simulink model "sdrzfreqcalib_rx"  (R2016a)
settings: Solver=FixedStepDiscrete  StartTime=0.0  StopTime=inf  RelTol=1e-3
libraries: sdrzblksprivate x1, dspspect3 x1, sdrzlib x1
Description:
  | This model is used to calculate the frequency offset between a transmitter and the SDR receiver.
settings Model: ModifiedByFormat=The MathWorks Inc.  SimulationMode=accelerator  Creator=The MathWorks, Inc.  LastModifiedBy=The MathWorks Inc.
settings DataIOCC: LimitDataPoints=on  SaveFormat=Array
settings OptimizationCC: ExpressionDepthLimit=2147483647
settings DebuggingCC: UnderspecifiedInitializationDetection=Classic  MergeDetectMultiDrivingBlocksExec=none  SolverPrmCheckMsg=warning  ParameterPrecisionLossMsg=none  FcnCallInpInsideContextMsg=EnableAllAsWarning  AllowSymbolicDim=off  StateNameClashWarn=warning
settings HardwareCC: ProdBitPerPointer=32  ProdLargestAtomicFloat=None  ProdIntDivRoundTo=Undefined  ProdEndianess=Unspecified  ProdWordSize=32  ProdHWDeviceType=32-bit Generic  TargetBitPerPointer=64  TargetLongLongMode=on  TargetIntDivRoundTo=Zero  TargetEndianess=LittleEndian  TargetWordSize=64  TargetHWDeviceType=Generic->MATLAB Host Computer  ProdEqTarget=off
settings ModelReferenceCC: PropagateSignalLabelsOutOfModel=off
settings RTWCC: CustomSourceCode=|
  | #include<stdio.h>
  | #include<stdlib.h>
settings GRTTargetCC: CombineOutputUpdateFcns=off  GRTInterface=on
settings ConfigComp: CovModelRefEnable=Off  CovSFcnEnable=off

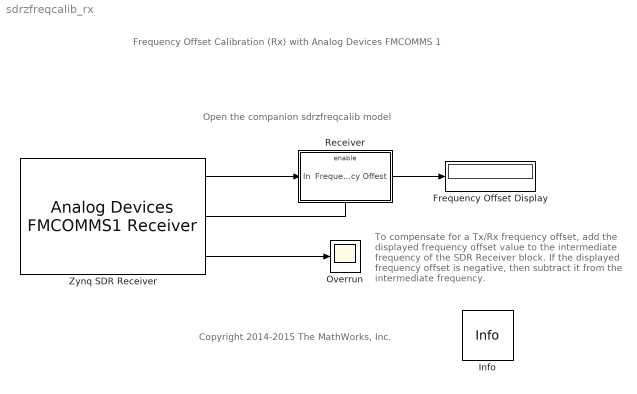
== system sdrzfreqcalib_rx ==
  note: Frequency Offset Calibration (Rx)
      | with Analog Devices FMCOMMS 1
  note: Open the companion sdrzfreqcalib model
  note: Copyright 2014-2015 The MathWorks, Inc.
  note: To compensate for a Tx/Rx frequency offset,
      | add the displayed frequency offset value to the
      | intermediate frequency of the SDR Receiver block. If
      | the displayed frequency offset is negative, then
      | subtract it from the intermediate frequency.
  Frequency Offset Display : Display
  Info : sdrzblksprivate/Info  SystemSampleTime=-1
  Overrun : Scope
  Receiver : Subsystem
      mask Display: disp('Receiver')
  Zynq SDR Receiver : sdrzlib/Analog Devices FMCOMMS1 Receiver  SourceLibraryInfo="This block requires Communications System Toolbox Support Package for Xilinx FPGA-Based Radio. <a href=\"http://www.mathworks.com/hardware-support-packages\">More information</a>"  sobjType=comm.SDRZynqFMCOMMS1Receiver  IPAddress=192.168.3.2  dataUDPPort=-1  ctrlUDPPort=-1  subDeviceList=comm.SDRZynqFMCOMMS1Receiver  sdrBlockType=SDRBlockTypeSLT.SDRRxBlock  requester=UNUSED_BY_SFCN  sdrExecutionMode=HW  LostSamplesOutputPort=on  OutputDataType=double  FrameLength=4096  EnableBurstMode=off  NumFramesInBurst=20  BypassUserLogic=on  DecimatorSelect=DDC decimator  SourceSelect=RF data  SineAmplitude=16000  SineFrequency=30000  EnableInternalClock=off  BypassIQBalance=on  CenterFrequencySource=Dialog  CenterFrequency=2.415e9 - 3e6  IntermediateFrequencySource=Dialog  IntermediateFrequency=3e6  IFBandwidthSource=Dialog  IFBandwidth=40e6  ADCRateSource=Dialog  ADCRate=98.304e6  GainSource=Dialog  Gain=4.5  DecimationFactorSource=Dialog  DecimationFactor=500  RFFrequencyIsTunable=logical(0)  SampleTime=1/(98.304e6/500)  BypassDCBlockingFilter=off  IQBalanceCoefficients=64  SkipAllHardwareResetAndInitialization=off  EnableIQCalibrationTable=on  CacheIQCalibrationTable=off
  wires:
  Zynq SDR Receiver/1 -> Receiver/1(In)
  Zynq SDR Receiver/2 -> Receiver/Enable
  Zynq SDR Receiver/3 -> Overrun/1
  Receiver/1(Frequency Offest) -> Frequency Offset Display/1

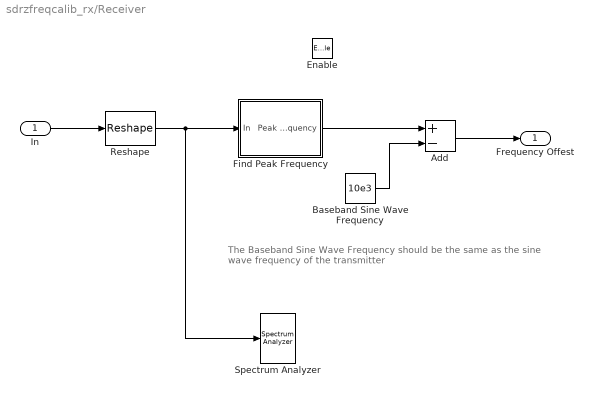
== system sdrzfreqcalib_rx/Receiver ==
  note: The Baseband Sine Wave Frequency should be the same as
      | the sine wave frequency of the transmitter
  In : Inport
  Enable : EnablePort
  Add : Sum  Inputs=+-
  Baseband Sine Wave Frequency : Constant  Value=10e3
  Find Peak Frequency : Subsystem
      mask Display: disp('Find Peak\nFrequency')
  Reshape : Reshape  OutputDimensionality=Customize  OutputDimensions=[4096,1]
  Spectrum Analyzer : SpectrumAnalyzer
  Frequency Offest : Outport
  wires:
  In/1 -> Reshape/1
  Reshape/1 -> Find Peak Frequency/1(In), Spectrum Analyzer/1
  Find Peak Frequency/1(Peak Frequency) -> Add/1
  Baseband Sine Wave Frequency/1 -> Add/2
  Add/1 -> Frequency Offest/1

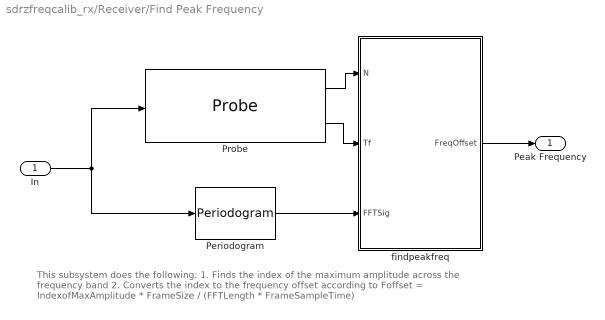
== system sdrzfreqcalib_rx/Receiver/Find Peak Frequency ==
  note: This subsystem does the following:
      | 1.  Finds the index of the maximum amplitude across the frequency band
      | 2.  Converts the index to the frequency offset according to
      | Foffset = IndexofMaxAmplitude * FrameSize / (FFTLength * FrameSampleTime)
  In : Inport
  Periodogram : dspspect3/Periodogram  measurement=Power spectral density  wintype=Hamming  Rs=50  beta=5  winsamp=Symmetric  FFTImplementation=Auto  inheritFFT=off  fftsize=4096  navg=2  inheritTs=on  Ts=1
  Probe : Probe  ProbeComplexSignal=off
  findpeakfreq : MATLAB Function  TreatAsAtomicUnit=on
  Peak Frequency : Outport
  wires:
  Periodogram/1 -> findpeakfreq/3(FFTSig)
  Probe/1 -> findpeakfreq/1(N)
  Probe/2 -> findpeakfreq/2(Tf)
  findpeakfreq/1(FreqOffset) -> Peak Frequency/1
  In/1 -> Periodogram/1, Probe/1

== matlab function sdrzfreqcalib_rx/Receiver/Find Peak Frequency/findpeakfreq ==
  data: N input; FreqOffset output; Tf input; FFTSig input
function FreqOffset  = findpeakfreq(N, Tf, FFTSig)
% Find peak frequency
% N - frame size
% Tf - frame sample time
% FFTSig - result of FFT

%#codegen

FFTSize = length(FFTSig);
FFTSig = fftshift(FFTSig);
[~, maxIdx] = max(FFTSig); % Find index of max magnitude
OffsetIdx = maxIdx-1-FFTSize/2; % Convert to index symmetric with 0
Ts = Tf(1)/N; % Sample time
delta_f = 1/Ts/FFTSize; % Frequency resolution of FFT
FreqOffset = OffsetIdx*delta_f;% Map offset index back to frequency
